simulink model "Control_Schematic_4"  (Simulink 8.3)
settings: Solver=FixedStepDiscrete  StartTime=0.0  StopTime=386.832  FixedStep=Ts  RelTol=1e-3
values from neighbouring files (symbols this model uses):
  B = [0 Kappa]'    [StartUp_5.m]    (also in StartUp_6.m)
  b = 156    [StartUp_10_Validation.m]    (also in StartUp_12.m; StartUp_12a.m; StartUp_2.m; StartUp_5.m)
  d = 13.52    [StartUp_10_Validation.m]    (also in StartUp_12.m; StartUp_12a.m; StartUp_2.m = 16.4; StartUp_5.m = 0.91)
  d0 = d*h    (= 0.328)    [StartUp_2.m]    (also in StartUp_5.m = 0.000455; StartUp_6.m = 0.000455)
  h = .02    (= 0.02)    [StartUp_2.m]    (also in StartUp_5.m = 0.0005; StartUp_6.m = 0.0005)
  K1 = .23    (= 0.23)    [StartUp_12.m]    (also in StartUp_12a.m; StartUp_2.m = PolyCon(1,2); StartUp_5.m = 16; StartUp_6.m = 16)
  K2 = .83    (= 0.83)    [StartUp_12.m]    (also in StartUp_12a.m; StartUp_2.m = 0.7; StartUp_5.m = 8; StartUp_6.m = 8)
  Kappa = (1E3/r)/((jw/r)+(m*r*.4))    (= 0.770469447034)    [StartUp_10_Validation.m]    (also in StartUp_12.m; StartUp_12a.m; StartUp_5.m = 0.000542967645047; StartUp_6.m = 0.000542967645047)
  Obz = c2d(Obs,Ts,'tustin')    [StartUp_2.m]    (also in StartUp_5.m; StartUp_6.m)
  P = [L(1,1) L(2,1);L(3,1) L(4,1)]    [StartUp_5.m]    (also in StartUp_6.m; charatioass.m = roots(K))
  r = 50    [StartUp_10_Validation.m]    (also in StartUp_12.m; StartUp_12a.m; StartUp_2.m = 820; StartUp_5.m = 0.01)
  R = 50    [StartUp_2.m]    (also in StartUp_5.m; StartUp_6.m)
  TD = ss(Atd,Btd,Ctd,Dtd,Ts)    [StartUp_12.m]    (also in StartUp_12a.m; StartUp_2.m; StartUp_5.m; StartUp_6.m)
  Ts = 1/100    (= 0.01)    [StartUp_10_Validation.m]    (also in StartUp_12.m; StartUp_12a.m; StartUp_2.m = 0.001; StartUp_5.m = 0.001)
undefined symbols (not defined in the file or in its folder): DiscIntNeverNeededParam, sigbuilder_block
undefined symbols (not defined in the file): ADAMS_cwd, ADAMS_exec, ADAMS_host, ADAMS_init, ADAMS_inputs, ADAMS_outputs, ADAMS_prefix, ADAMS_static, ADAMS_sysdir
libraries: simulink x1
settings Model: Creator=baqumau  LastModifiedBy=baqumau
settings DataIOCC: SignalLoggingSaveFormat=Dataset
settings DebuggingCC: UnderspecifiedInitializationDetection=Simplified  StateNameClashWarn=none
settings GRTTargetCC: CombineOutputUpdateFcns=on  GRTInterface=off

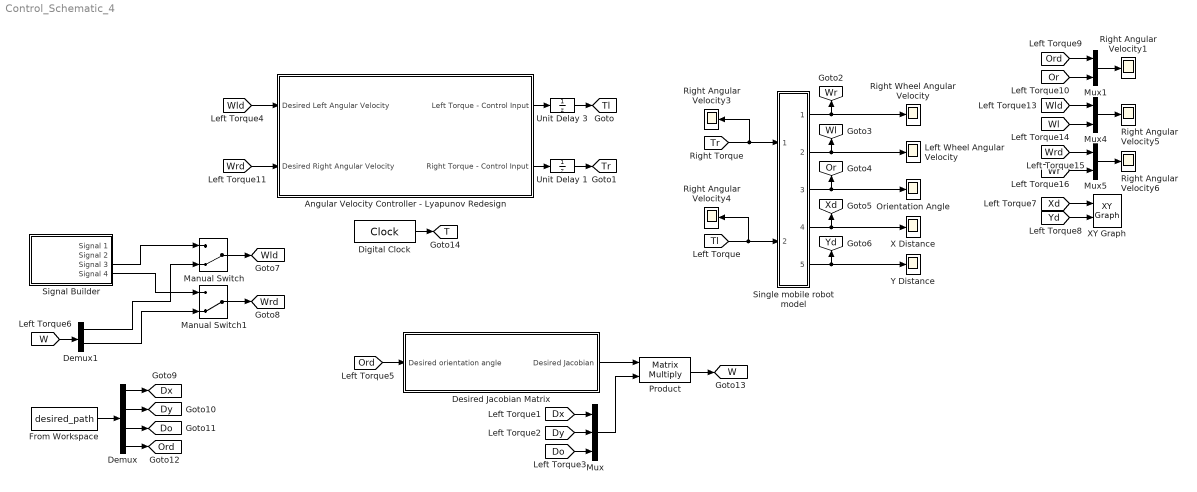
== system Control_Schematic_4 ==
  Angular Velocity Controller - Lyapunov Redesign : Subsystem
  Demux : Demux
  Demux1 : Demux  Outputs=2
  Desired Jacobian Matrix : Subsystem
  Digital Clock : DigitalClock  SampleTime=Ts
  From Workspace : FromWorkspace  VariableName=desired_path  SampleTime=Ts
  Left Wheel Angular Velocity : Scope
      settings: SaveName=ScopeData2
  Manual Switch : ManualSwitch  CurrentSetting=0
  Manual Switch1 : ManualSwitch  CurrentSetting=0
  Mux : Mux  Inputs=3
  Mux1 : Mux  Inputs=2
  Mux4 : Mux  Inputs=2
  Mux5 : Mux  Inputs=2
  Orientation Angle : Scope
      settings: YMin=-4  YMax=4
  Product : Product  Multiplication=Matrix(*)
  Right Angular Velocity{1,3..6} (5 alike) : Scope
      Right Angular Velocity1 settings: YMin=-3  YMax=3  SaveName=ScopeData27
      Right Angular Velocity3 settings: YMin=-25  YMax=25  SaveName=ScopeData7
      Right Angular Velocity4 settings: YMin=-25  YMax=25  SaveName=ScopeData8
      Right Angular Velocity5 settings: YMin=-1  YMax=1  SaveName=ScopeData9
      Right Angular Velocity6 settings: YMin=-1  YMax=3  SaveName=ScopeData10
  Right Wheel Angular Velocity : Scope
      settings: YMin=-1  YMax=1  SaveName=ScopeData3
  Signal Builder : Subsystem  Tag=STV Subsys  LoadFcn=sigbuilder_block('load');  StartFcn=sigbuilder_block('start');  StopFcn=sigbuilder_block('stop');  ClipboardFcn=sigbuilder_block('clipboard');  mask(Sigbuilder block){}
      mask help: Simulink:masks:SigbuilderBlock_MD
      mask init:
      | if ~strcmp(get_param(bdroot(gcbh),'SimulationStatus'),'stopped') tuvar = sigbuilder_block('maskInit'); end
      settings: CopyFcn=sigbuilder_block('copy');  DeleteFcn=sigbuilder_block('delete');  ModelCloseFcn=sigbuilder_block('modelClose');  PreSaveFcn=sigbuilder_block('preSave');  PauseFcn=sigbuilder_block('pause');  ContinueFcn=sigbuilder_block('continue');  NameChangeFcn=sigbuilder_block('namechange');  OpenFcn=sigbuilder_block('open',[437.25 118.5 550.5 394.5 ]);  CloseFcn=sigbuilder_block('close');
      mask Display: plot(0, 0, 100, 100,[2, 2, 32, 32, 2], [68, 8, 8, 68, 68],[32, 2], [38, 38], [32, 19, 2],[53, 60, 44], [32, 17, 17, 2],[16, 16, 31, 31]);txt = getActiveGroup(gcbh);text(2, 100, txt,'verticalAlignment', 'top');
  Single mobile robot model : Subsystem
  Unit Delay 1 : UnitDelay  SampleTime=-1
  Unit Delay 3 : UnitDelay  SampleTime=-1
  X Distance : Scope
      settings: YMin=0  YMax=2600  SaveName=ScopeData4
  XY Graph : simulink/Sinks/XY Graph  xmin=0  xmax=5000  ymin=0  ymax=5000  st=Ts
  Y Distance : Scope
      settings: YMin=0  YMax=1000
  tag scope: Do=global, Dx=global, Dy=global, Or=global, Ord=global, T=global, Tl=global, Tr=global, W=global, Wl=global, Wld=global, Wr=global, Wrd=global, Xd=global, Yd=global
  wires:
  Single mobile robot model/1(Wrw) -> Right Wheel Angular Velocity/1, [Wr]
  Single mobile robot model/2(Wlw) -> Left Wheel Angular Velocity/1, [Wl]
  Single mobile robot model/3(Alpha) -> Orientation Angle/1, [Or]
  Single mobile robot model/4(X_Dist) -> X Distance/1, [Xd]
  Single mobile robot model/5(Y_Dist) -> Y Distance/1, [Yd]
  [Tr] -> Single mobile robot model/1(Trw), Right Angular Velocity3/1
  [Tl] -> Single mobile robot model/2(Tlw), Right Angular Velocity4/1
  [Wld] -> Angular Velocity Controller - Lyapunov Redesign/1(Desired Left Angular Velocity)
  [Wrd] -> Angular Velocity Controller - Lyapunov Redesign/2(Desired Right Angular Velocity)
  [Wld] -> Mux4/1
  [Wl] -> Mux4/2
  Mux4/1 -> Right Angular Velocity5/1
  [Wrd] -> Mux5/1
  [Wr] -> Mux5/2
  Mux5/1 -> Right Angular Velocity6/1
  Manual Switch/1 -> [Wld]
  Manual Switch1/1 -> [Wrd]
  From Workspace/1 -> Demux/1
  Demux/1 -> [Dx]
  Demux/2 -> [Dy]
  Demux/3 -> [Do]
  Demux/4 -> [Ord]
  [Dy] -> Mux/2
  [Dx] -> Mux/1
  [Do] -> Mux/3
  [Ord] -> Desired Jacobian Matrix/1(Desired orientation angle)
  Desired Jacobian Matrix/1(Desired Jacobian) -> Product/1
  Mux/1 -> Product/2
  Product/1 -> [W]
  [W] -> Demux1/1
  Demux1/1 -> Manual Switch/2
  Demux1/2 -> Manual Switch1/2
  Signal Builder/3(Signal 3) -> Manual Switch/1
  Signal Builder/4(Signal 4) -> Manual Switch1/1
  [Xd] -> XY Graph/1
  [Yd] -> XY Graph/2
  Digital Clock/1 -> [T]
  [Ord] -> Mux1/1
  [Or] -> Mux1/2
  Mux1/1 -> Right Angular Velocity1/1
  Angular Velocity Controller - Lyapunov Redesign/1(Left Torque - Control Input) -> Unit Delay 3/1
  Angular Velocity Controller - Lyapunov Redesign/2(Right Torque - Control Input) -> Unit Delay 1/1
  Unit Delay 3/1 -> [Tl]
  Unit Delay 1/1 -> [Tr]

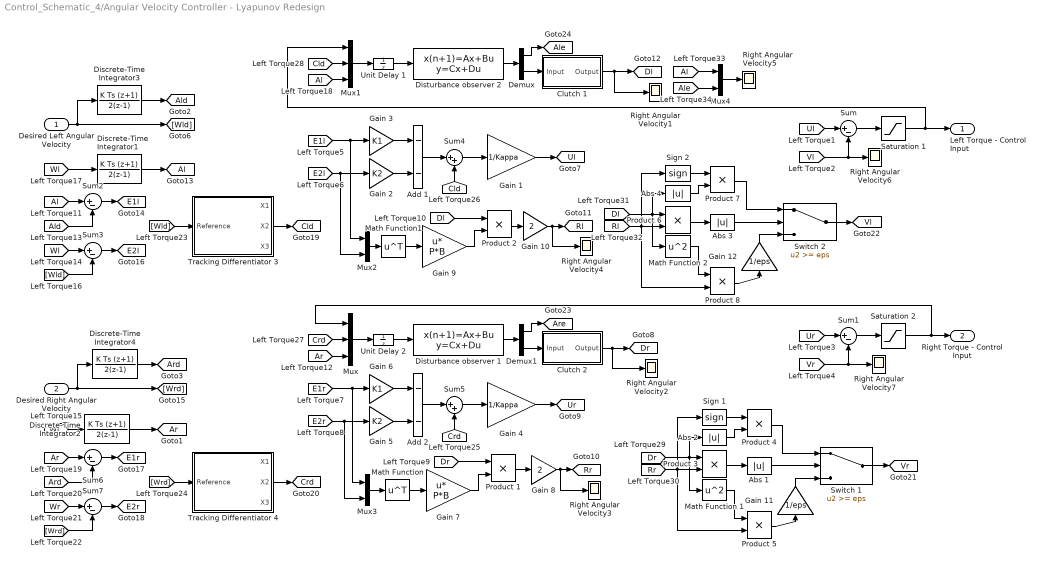
== system Control_Schematic_4/Angular Velocity Controller - Lyapunov Redesign ==
  Desired Left Angular Velocity : Inport
  Desired Right Angular Velocity : Inport  Port=2
  Abs {1..4} (4 alike) : Abs
  Add 1 : Sum  Inputs=--
  Add 2 : Sum  Inputs=--
  Clutch 1 : Subsystem
  Clutch 2 : Subsystem
  Demux : Demux  Outputs=2
  Demux1 : Demux  Outputs=2
  Discrete-Time Integrator{1..4} (4 alike) : DiscreteIntegrator  IntegratorMethod=Integration: Trapezoidal  gainval=1  SampleTime=Ts  ICPrevOutput=DiscIntNeverNeededParam  ICPrevScaledInput=DiscIntNeverNeededParam
  Disturbance observer 1 : DiscreteStateSpace  A=Obz.a  B=Obz.b  C=Obz.c  D=Obz.d  SampleTime=Ts
  Disturbance observer 2 : DiscreteStateSpace  A=Obz.a  B=Obz.b  C=Obz.c  D=Obz.d  SampleTime=Ts
  Gain 1 : Gain  Gain=1/Kappa
  Gain 10 : Gain  Gain=2
  Gain 11 : Gain  Gain=1/eps
  Gain 12 : Gain  Gain=1/eps
  Gain 2 : Gain  Gain=K2
  Gain 3 : Gain  Gain=K1
  Gain 4 : Gain  Gain=1/Kappa
  Gain 5 : Gain  Gain=K2
  Gain 6 : Gain  Gain=K1
  Gain 7 : Gain  Gain=P*B  Multiplication=Matrix(u*K)
  Gain 8 : Gain  Gain=2
  Gain 9 : Gain  Gain=P*B  Multiplication=Matrix(u*K)
  Math Function : Math  Operator=transpose  SaturateOnIntegerOverflow=on
  Math Function 1 : Math  Operator=square  SaturateOnIntegerOverflow=on
  Math Function 2 : Math  Operator=square  SaturateOnIntegerOverflow=on
  Math Function1 : Math  Operator=transpose  SaturateOnIntegerOverflow=on
  Mux : Mux  Inputs=3
  Mux1 : Mux  Inputs=3
  Mux2 : Mux  Inputs=2
  Mux3 : Mux  Inputs=2
  Mux4 : Mux  Inputs=2
  Product {1..8} (8 alike) : Product
  Right Angular Velocity{1..7} (7 alike) : Scope
      Right Angular Velocity1 settings: YMin=-3  YMax=3  SaveName=ScopeData5
      Right Angular Velocity2 settings: YMin=-3  YMax=3  SaveName=ScopeData6
      Right Angular Velocity3 settings: YMin=-3  YMax=3  SaveName=ScopeData11
      Right Angular Velocity4 settings: YMin=-3  YMax=3  SaveName=ScopeData12
      Right Angular Velocity5 settings: YMin=-1  YMax=1  SaveName=ScopeData13
      Right Angular Velocity6 settings: YMin=-3  YMax=3  SaveName=ScopeData14
      Right Angular Velocity7 settings: YMin=-3  YMax=3  SaveName=ScopeData15
  Saturation 1 : Saturate  UpperLimit=20  LowerLimit=-20
  Saturation 2 : Saturate  UpperLimit=20  LowerLimit=-20
  Sign 1 : Signum
  Sign 2 : Signum
  Sum{,1..3,6..7} (6 alike) : Sum  Inputs=|+-
  Sum4 : Sum  Inputs=|++
  Sum5 : Sum  Inputs=|++
  Switch 1 : Switch  Threshold=eps
  Switch 2 : Switch  Threshold=eps
  Tracking Differentiator 3 : Subsystem
  Tracking Differentiator 4 : Subsystem
  Unit Delay 1 : UnitDelay  SampleTime=-1
  Unit Delay 2 : UnitDelay  SampleTime=-1
  Left Torque - Control Input : Outport
  Right Torque - Control Input : Outport  Port=2
  tag scope: Al=global, Ald=global, Ale=global, Ar=global, Ard=global, Are=global, Cld=global, Crd=global, Dl=global, Dr=global, E1l=global, E1r=global, E2l=global, E2r=global, Rl=global, Rr=global, Ul=global, Ur=global, Vl=global, Vr=global
  wires:
  Discrete-Time Integrator1/1 -> [Al]
  Discrete-Time Integrator2/1 -> [Ar]
  Saturation 1/1 -> Mux1/1, Left Torque - Control Input/1
  Saturation 2/1 -> Mux/1, Right Torque - Control Input/1
  Discrete-Time Integrator4/1 -> [Ard]
  Discrete-Time Integrator3/1 -> [Ald]
  [Wl] -> Discrete-Time Integrator1/1
  [Wr] -> Discrete-Time Integrator2/1
  Mux/1 -> Unit Delay 2/1
  Mux1/1 -> Unit Delay 1/1
  Sum/1 -> Saturation 1/1
  Sum1/1 -> Saturation 2/1
  [Ul] -> Sum/1
  [Ur] -> Sum1/1
  Gain 3/1 -> Add 1/1
  Gain 2/1 -> Add 1/2
  Gain 1/1 -> [Ul]
  Gain 6/1 -> Add 2/1
  Gain 5/1 -> Add 2/2
  [E1r] -> Mux3/1, Gain 6/1
  [E2r] -> Mux3/2, Gain 5/1
  Gain 4/1 -> [Ur]
  [Dr] -> Product 1/1
  Mux3/1 -> Math Function/1
  [E1l] -> Mux2/1, Gain 3/1
  [E2l] -> Mux2/2, Gain 2/1
  [Al] -> Sum2/1
  [Ald] -> Sum2/2
  Sum2/1 -> [E1l]
  [Wl] -> Sum3/1
  [Wld] -> Sum3/2
  Sum3/1 -> [E2l]
  Sum4/1 -> Gain 1/1
  Sum5/1 -> Gain 4/1
  [Ar] -> Sum6/1
  [Ard] -> Sum6/2
  Sum6/1 -> [E1r]
  [Wr] -> Sum7/1
  [Wrd] -> Sum7/2
  Sum7/1 -> [E2r]
  Add 2/1 -> Sum5/1
  Add 1/1 -> Sum4/1
  [Wld] -> Tracking Differentiator 3/1(Reference)
  Tracking Differentiator 3/2(X2) -> [Cld]
  [Wrd] -> Tracking Differentiator 4/1(Reference)
  Tracking Differentiator 4/2(X2) -> [Crd]
  [Ar] -> Mux/3
  [Crd] -> Mux/2
  [Al] -> Mux1/3
  [Cld] -> Mux1/2
  [Dr] -> Math Function 1/1, Abs 2/1, Product 3/1
  [Rr] -> Product 5/2, Sign 1/1, Product 3/2
  Product 3/1 -> Abs 1/1
  Abs 1/1 -> Switch 1/2
  Switch 1/1 -> [Vr]
  Sign 1/1 -> Product 4/1
  Abs 2/1 -> Product 4/2
  Product 4/1 -> Switch 1/1
  Math Function 1/1 -> Product 5/1
  Product 5/1 -> Gain 11/1
  Gain 11/1 -> Switch 1/3
  [Dl] -> Product 6/1, Abs 4/1, Math Function 2/1
  [Rl] -> Product 6/2, Sign 2/1, Product 8/2
  Product 6/1 -> Abs 3/1
  Abs 3/1 -> Switch 2/2
  Switch 2/1 -> [Vl]
  Sign 2/1 -> Product 7/1
  Abs 4/1 -> Product 7/2
  Product 7/1 -> Switch 2/1
  Math Function 2/1 -> Product 8/1
  Product 8/1 -> Gain 12/1
  Gain 12/1 -> Switch 2/3
  Math Function/1 -> Gain 7/1
  Gain 7/1 -> Product 1/2
  Product 1/1 -> Gain 8/1
  Gain 8/1 -> Right Angular Velocity3/1, [Rr]
  [Dl] -> Product 2/1
  Math Function1/1 -> Gain 9/1
  Gain 9/1 -> Product 2/2
  Product 2/1 -> Gain 10/1
  Mux2/1 -> Math Function1/1
  Unit Delay 1/1 -> Disturbance observer 2/1
  Unit Delay 2/1 -> Disturbance observer 1/1
  Gain 10/1 -> Right Angular Velocity4/1, [Rl]
  Clutch 1/1(Output) -> Right Angular Velocity1/1, [Dl]
  Clutch 2/1(Output) -> Right Angular Velocity2/1, [Dr]
  Disturbance observer 2/1 -> Demux/1
  Demux/2 -> Clutch 1/1(Input)
  Disturbance observer 1/1 -> Demux1/1
  Demux1/2 -> Clutch 2/1(Input)
  Demux1/1 -> [Are]
  Demux/1 -> [Ale]
  [Ale] -> Mux4/2
  Mux4/1 -> Right Angular Velocity5/1
  [Al] -> Mux4/1
  [Vr] -> Right Angular Velocity7/1, Sum1/2
  [Vl] -> Right Angular Velocity6/1, Sum/2
  [Cld] -> Sum4/2
  [Crd] -> Sum5/2
  Desired Left Angular Velocity/1 -> [Wld], Discrete-Time Integrator3/1
  Desired Right Angular Velocity/1 -> [Wrd], Discrete-Time Integrator4/1

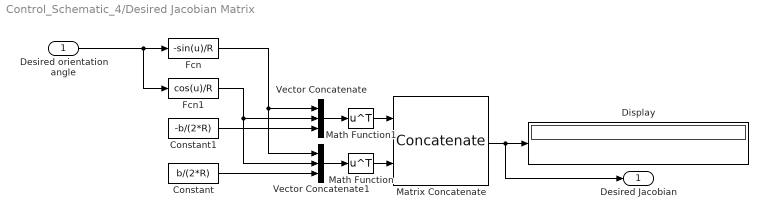
== system Control_Schematic_4/Desired Jacobian Matrix ==
  Desired orientation angle : Inport
  Constant : Constant  Value=b/(2*R)
  Constant1 : Constant  Value=-b/(2*R)
  Display : Display
  Fcn : Fcn  Expr=-sin(u)/R
  Fcn1 : Fcn  Expr=cos(u)/R
  Math Function : Math  Operator=transpose  SaturateOnIntegerOverflow=on
  Math Function1 : Math  Operator=transpose  SaturateOnIntegerOverflow=on
  Matrix Concatenate : Concatenate  Mode=Multidimensional array
  Vector Concatenate : Concatenate  NumInputs=3
  Vector Concatenate1 : Concatenate  NumInputs=3
  Desired Jacobian : Outport
  wires:
  Math Function/1 -> Matrix Concatenate/2
  Math Function1/1 -> Matrix Concatenate/1
  Desired orientation angle/1 -> Fcn1/1, Fcn/1
  Constant1/1 -> Vector Concatenate/3
  Matrix Concatenate/1 -> Desired Jacobian/1, Display/1
  Fcn/1 -> Vector Concatenate1/1, Vector Concatenate/1
  Vector Concatenate/1 -> Math Function1/1
  Fcn1/1 -> Vector Concatenate1/2, Vector Concatenate/2
  Constant/1 -> Vector Concatenate1/3
  Vector Concatenate1/1 -> Math Function/1

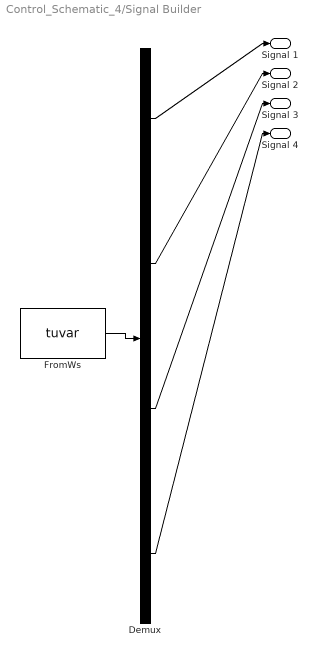
== system Control_Schematic_4/Signal Builder ==
  Demux : Demux  Tag=STV Demux
  FromWs : FromWorkspace  Tag=STV FromWs  VariableName=tuvar  SampleTime=0  SigBuilderData=DataTag0  VnvData=DataTag1
      SigBuilderData=|
      | common.afterFinalStr = 'Extrapolate'
      | common.sampleTime = 0
      | dataSet.timeRange = [0 10]
      | dataSet.name = 'Group 1'
      | sbobj.Groups.Name = 'Group 1'
      | sbobj.Groups.Signals(1).Name = 'Signal 1'
      | sbobj.Groups.Signals(1).XData = [0 1 2 3 4 5 6 7 8 8 9 10]
      | sbobj.Groups.Signals(1).YData = [0 1.5 2.05 1.54 0.9 0 -1.58 -2.05 -1.65 -1.66 0 0.85]
      | sbobj.Groups.Signals(2).Name = 'Signal 2'
      | sbobj.Groups.Signals(2).XData = [0 1 2 2 3 4 4 5 6 7 8 9 10]
      | sbobj.Groups.Signals(2).YData = [0 -1 -1.35 -1.3 -2 -2 -2.05 -0.6 2 2 1.5 -1.15 -2.85]
      | sbobj.Groups.Signals(3).Name = 'Signal 3'
      | sbobj.Groups.Signals(3).XData = [0 10]
      | sbobj.Groups.Signals(3).YData = [1.28205128205 1.28205128205]
      | sbobj.Groups.Signals(4).Name = 'Signal 4'
      | sbobj.Groups.Signals(4).XData = [0 10]
      | sbobj.Groups.Signals(4).YData = [0 0]
  Signal 1 : Outport  Tag=STV Outport
  Signal 2 : Outport  Tag=STV Outport  Port=2
  Signal 3 : Outport  Tag=STV Outport  Port=3
  Signal 4 : Outport  Tag=STV Outport  Port=4
  wires:
  FromWs/1 -> Demux/1
  Demux/1 -> Signal 1/1
  Demux/2 -> Signal 2/1
  Demux/3 -> Signal 3/1
  Demux/4 -> Signal 4/1

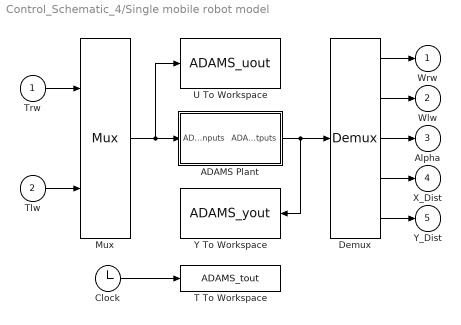
== system Control_Schematic_4/Single mobile robot model ==
  Trw : Inport
  Tlw : Inport  Port=2
  ADAMS Plant : Subsystem  LoadFcn=|  InitFcn=clear mex  mask(Adams Plant){exevie=ADAMS_sysdir, nam_in=ADAMS_inputs, namout=ADAMS_outputs, nampre=ADAMS_prefix, outfil=ADAMS_prefix, exesol=ADAMS_exec, stat=ADAMS_static, inicmd=[ADAMS_init], exetyp=C++, comtyp=PIPE(DDE), workdir=ADAMS_cwd, ada_host=ADAMS_host, modani=batch, modsim=discrete, dft=no, simulink_lead_cosim=yes, pin_interp_order=0, pout_extrap_order=0, pin_extrap_order=0, pout_interp_order=0, dt_out=Ts, o_rate=1, more=off}
      | %check based on dialog box setting for when setting by popup menu                                             
      | if exist('ADAMS_solver_type')                                                                                 
      |   if strcmp(ADAMS_solver_type,'C++')                                                                          
      |     set_param(gcb,'exetyp','C++');                                                                            
      |   else                                                                                                        
      |     set_param(gcb,'exetyp','Fortran');                                                                        
      |   end                                                                                                         
      | else                                                                                                          
      |   set_param(gcb,'exetyp','C++');                                                                              
      | end                                                                                                           
      | %set the mode if using acar_solver                                                                            
      | %REQUIRED HERE BECAUSE BELOW CAUSES MDLTERMINATE TO BE CALLED 2 TIMES IN MIDDLE OF SIMULATION WHEN SET IN MASK
      |                                                                                                               
      | %enable the direct feedthrough, sim mode, anim mode parameters by default                                     
      |                                                                                                               
      | if exist('set_some_params_states')                                                                            
      |                                                                                                               
      |   set_some_params_states({'dft','modsim','modani'},{'on','on','on'},'MaskEnables',gcb)                        
      |   %turn on direct feedthrough option                                                                          
      |   set_some_params_states({'dft'},{'on'},'MaskVisibilities',gcb)                                               
      |                                                                                                               
      |  end                                                                                                          
      |                                                                                                               
      |                                                                                                               
      | if exist('ADAMS_exec')                                                                                        
      |   if and(strcmp(get_param(gcb,'exesol'),'ADAMS_exec'),strcmp(ADAMS_exec,'acar_solver'))                       
      |     %set the sim mode to discrete -- only supported mode                                                      
      |     set_param(gcb,'modsim','discrete')                                                                        
      |      %turn off direct feedthrough option                                                                      
      |      set_some_params_states({'dft'},{'off'},'MaskVisibilities',gcb)                                           
      |     %set the animation mode to batch -- only supported mode                                                   
      |     set_param(gcb,'modani','batch')                                                                           
      |     %disable the direct feedthrough, sim mode, anim mode parameters                                           
      |     set_some_params_states({'modsim','modani'},{'off','off'},'MaskEnables',gcb)                               
      |   end                                                                                                         
      | end
      mask prompts: exevie "Adams install directory"; nam_in "Adams/View input names"; namout "Adams/View output names"; nampre "Adams model file prefix"; outfil "Output files prefix (opt.: if blank - no output)"; exesol "User executable (opt.: if blank - use standard)"; stat "Initial static simulation flag"; inicmd "Initialization commands"; exetyp "Adams/Solver type"; comtyp "Interprocess option"; workdir "Adams working directory"; ada_host "Adams host"; modani "Animation mode"; modsim "Simulation mode"; dft "Direct feedthrough"; simulink_lead_cosim "Discrete Computational Order - Simulink Leads Adams"; pin_interp_order "Plant input interpolation order"; pout_extrap_order "Plant output extrapolation order"; pin_extrap_order "Plant input extrapolation order"; pout_interp_order "Plant output interpolation order"; dt_out "Communication interval"; o_rate "Number of communications per output step"; more "More parameters"
      mask help: Simulate any Adams plant model either in Adams/Solver form (.adm file) or in Adams/View form (.cmd file)
      settings: OpenFcn=|
      | open_system(gcb,'mask')
      | if not(exist('set_some_params_states'))
      | 
      | warning('The script "set_some_params_states.m" cannot be found in the MATLAB PATH.  Cannot update the ADAMS Plant S-Function parameters.')
      | 
      | warning('Recommended action(optional):  run the Adams/Controls .m file first to help choose the correct settings in the Adams S-Function block.')
      | 
      | end
      mask Help:
      | <html>
      | This S-Function represents the non-linear Adams Plant with the inputs sent to the Adams model <br>
      |  and the outputs generated by the Adams model.  See the Adams/Controls documentation for more <br>
      | information.  This plant uses the following variables:<br>
      | <br>
      | <b>ADAMS_sysdir  :</b> Adams installation directory<br>
      | <b>ADAMS_inputs  :</b> Input variables View names vector<br>
      | <b>ADAMS_outputs :</b> Outputs variables View names vector<br>
      | <b>ADAMS_prefix  : </b>ADAMS model files prefix (.adm, .cmd); also doubles as output files prefix<br>
      | <b>ADAMS_exec :</b> Adams/Solver user library or keyword (e.g., acar_solver)<br>
      | <b>ADAMS_static :</b> yes|no - initial static before Co-simulation(discrete)/Function Evaluation(continuous)<br>
      | <b>ADAMS_init :</b>Initialization commands (i.e., Adams/View or Solver commands, depending on setting for Animation mode)<br>
      | <b>ADAMS_cwd : </b> Current working directory (for TCP/IP)<br>
      | <b>ADAMS_host : </b>Name of Adams server host (for TCP/IP)<br>
      | <b>ADAMS_mode :</b> Linear or non-linear (i.e., co-sim, function eval)<br>
      | <b>ADAMS_solver_type :</b>Fortran or C++ (used to set popup menu when first loaded) <br>
      | 
      | 
      | <br>
      | The following settings can be chosen:<br>
      | <br>
      | <b>Adams/Solver type:</b>  Fortran or C++ (will also set ADAMS_solver_type)<br>
      | <b>Interprocess option:</b> Pipe(DDE) or TCP/IP; TCP/IP can allow different machines run Adams and MATLAB<br>
      | <b>Animation mode:</b> batch (Solver, uses .adm) or interactive (View, uses .cmd)<br>
      | <b>Simulation mode:</b> discrete (Co-simulation) or continuous (Function Evaluation)<br>
      | <b>Discrete Computational Order - Simulink Lead Adams:</b> for discrete mode, chooses if Simulink leads the integration (yes) or lags (no);<br> if set to "no", can remove algebraic loop<br>
      | <b>Plant input interpolation order:</b> 0 = zero-order hold; 1 = linear (discrete mode only, where Simulink leads)<br>
      | <b>Plant output extrapolation order:</b> 0 = zero-order hold;1 = linear(discrete mode only, where Simulink leads)<br>
      | <b>Plant input extrapolation order:</b> 0 = zero-order hold; 1 = linear (discrete mode only, where Adams leads)<br>
      | <b>Plant output interpolation order:</b> 0 = zero-order hold;1 = linear(discrete mode only, where Adams leads)<br>
      | <b>Direct feedthrough:</b> yes|no - yes = Input directly effect output(continuous mode-only)<br>
      | <b>Communication interval:</b> Time step at which Co-simulation exchange information (e.g.,0.005); also controls <br>output for continuous mode (Function Evaluation)<br>
      | <b>Number of communications per output step: </b>Sets Adams output rate (.res, .req, .gra) integer value (default: 1)<br>
      | </html>
      mask Callback exesol:
      | if exist('set_some_params_states')
      | %enable the direct feedthrough, sim mode, anim mode parameters
      | set_some_params_states({'dft','modsim','modani'},{'on','on','on'},'MaskEnables',gcb)
      | %turn on direct feedthrough option
      | set_some_params_states({'dft'},{'on'},'MaskVisibilities',gcb)
      | end
      | 
      | if exist('ADAMS_exec')
      |   if and(strcmp(get_param(gcb,'exesol'),'ADAMS_exec'),strcmp(ADAMS_exec,'acar_solver'))
      |     %set the sim mode to discrete -- only supported mode
      |     %REMOVED:  BELOW CAUSES MDLTERMINATE TO BE CALLED 2 TIMES IN MIDDLE OF SIMULATION
      |     %Now in LoadFcn callback
      |     %set_param(gcb,'modsim','discrete')
      |      %turn off direct feedthrough option
      |     set_some_params_states({'dft'},{'off'},'MaskVisibilities',gcb)
      |     %set the animation mode to batch -- only supported mode
      |     %REMOVED:  BELOW CAUSES MDLTERMINATE TO BE CALLED 2 TIMES IN MIDDLE OF SIMULATION
      |     %Now in LoadFcn callback
      |     %set_param(gcb,'modani','batch')
      |     %disable the direct feedthrough, sim mode, anim mode parameters
      |     set_some_params_states({'modsim','modani'},{'off','off'},'MaskEnables',gcb)
      |   end
      | end
      mask TypeOptions exetyp: Fortran | C++
      mask Callback exetyp:
      | if strcmp(get_param(gcb,'exetyp'),'C++')
      |     ADAMS_solver_type='C++';
      | else
      |     ADAMS_solver_type='Fortran';
      | end
      mask TypeOptions comtyp: PIPE(DDE) | TCP/IP
      mask Callback comtyp:
      | if exist('set_some_params_states')
      | if strcmp(get_param(gcb,'comtyp'),'PIPE(DDE)')
      |     %turn off cwd, host options
      |     set_some_params_states({'ada_host','workdir'},{'off','off'},'MaskVisibilities',gcb)
      | else%if strcmp(get_param(gcb,'modsim'),'TCP/IP')
      |     %turn on cwd, host options
      |     set_some_params_states({'ada_host','workdir'},{'on','on'},'MaskVisibilities',gcb)
      | end
      | end
      mask TypeOptions modani: batch | interactive
      mask TypeOptions modsim: discrete | continuous
      mask Callback modsim:
      | if exist('set_some_params_states')
      | if strcmp(get_param(gcb,'modsim'),'discrete')
      |      %turn off direct feedthrough option
      |     set_some_params_states({'dft'},{'off'},'MaskVisibilities',gcb)
      |     %turn on discrete co-sim type if want to see more
      |     if strcmp(get_param(gcb,'more'),'on')
      |         set_some_params_states({'simulink_lead_cosim'},{'on'},'MaskVisibilities',gcb)
      |     end
      |     if strcmp(get_param(gcb,'simulink_lead_cosim'),'yes')
      |         %turn on interpolation/extrapolation options
      |         set_some_params_states({'pin_interp_order','pout_extrap_order',},{'on','on'},'MaskVisibilities',gcb)
      |     else
      |         set_some_params_states({'pin_extrap_order','pout_interp_order'},{'on','on'},'MaskVisibilities',gcb)
      |     end
      | else%if strcmp(get_param(gcb,'modsim'),'continuous')
      |      %turn off direct feedthrough option
      |     set_some_params_states({'dft'},{'on'},'MaskVisibilities',gcb)
      |     %turn off interpolation/extrapolation options
      |     set_some_params_states({'pin_interp_order','pout_extrap_order','pin_extrap_order','pout_interp_order','simulink_lead_cosim'},{'off','off','off','off','off'},'MaskVisibilities',gcb)
      | end
      | end
      mask TypeOptions dft: no | yes
      mask TypeOptions simulink_lead_cosim: yes | no
      mask Callback simulink_lead_cosim:
      | if exist('set_some_params_states')
      | if (strcmp(get_param(gcb,'simulink_lead_cosim'),'yes') && strcmp(get_param(gcb,'modsim'),'discrete'))
      |      %turn off unused interpolate/extrapolate options
      |     set_some_params_states({'pin_extrap_order','pout_interp_order'},{'off','off'},'MaskVisibilities',gcb)
      |     %turn on used interpolate/extrapolate options
      |     set_some_params_states({'pin_interp_order','pout_extrap_order'},{'on','on'},'MaskVisibilities',gcb)
      | elseif (strcmp(get_param(gcb,'simulink_lead_cosim'),'no') && strcmp(get_param(gcb,'modsim'),'discrete'))
      |     %turn on used interpolate/extrapolate options
      |     set_some_params_states({'pin_extrap_order','pout_interp_order'},{'on','on'},'MaskVisibilities',gcb)
      |      %turn off unused interpolate/extrapolate options
      |     set_some_params_states({'pin_interp_order','pout_extrap_order'},{'off','off'},'MaskVisibilities',gcb)
      | end
      | end
      mask TypeOptions pin_interp_order: 0 | 1
      mask TypeOptions pout_extrap_order: 0 | 1
      mask TypeOptions pin_extrap_order: 0 | 1
      mask TypeOptions pout_interp_order: 0 | 1
      mask Callback more:
      | if exist('set_some_params_states')
      | if (strcmp(get_param(gcb,'more'),'on'))
      |      %turn on infrequently used options
      |     set_some_params_states({'exevie','nam_in','namout','exesol','stat','inicmd'},{'on','on','on','on','on','on'},'MaskVisibilities',gcb)
      |     if strcmp(get_param(gcb,'modsim'),'discrete')
      |         set_some_params_states({'simulink_lead_cosim'},{'on'},'MaskVisibilities',gcb)
      |     end
      | elseif (strcmp(get_param(gcb,'more'),'off'))
      |     %turn off infrequently used options
      |     set_some_params_states({'exevie','nam_in','namout','exesol','stat','inicmd'},{'off','off','off','off','off','off'},'MaskVisibilities',gcb)
      |     if strcmp(get_param(gcb,'modsim'),'discrete')
      |         set_some_params_states({'simulink_lead_cosim'},{'off'},'MaskVisibilities',gcb)
      |     end
      | end
      | end
      mask Display: disp( 'MSC Software' )
  Clock : Clock
  Demux : Demux  Outputs=5
  Mux : Mux  Inputs=2
  T To Workspace : ToWorkspace  VariableName=ADAMS_tout
      settings: MaxDataPoints=100000
  U To Workspace : ToWorkspace  VariableName=ADAMS_uout
      settings: MaxDataPoints=100000
  Y To Workspace : ToWorkspace  VariableName=ADAMS_yout
      settings: MaxDataPoints=100000
  Wrw : Outport
  Wlw : Outport  Port=2
  Alpha : Outport  Port=3
  X_Dist : Outport  Port=4
  Y_Dist : Outport  Port=5
  wires:
  Tlw/1 -> Mux/2
  Trw/1 -> Mux/1
  Demux/5 -> Y_Dist/1
  Demux/4 -> X_Dist/1
  Demux/3 -> Alpha/1
  Demux/2 -> Wlw/1
  Demux/1 -> Wrw/1
  ADAMS Plant/1(ADAMS outputs) -> Y To Workspace/1, Demux/1
  Mux/1 -> U To Workspace/1, ADAMS Plant/1(ADAMS inputs)
  Clock/1 -> T To Workspace/1

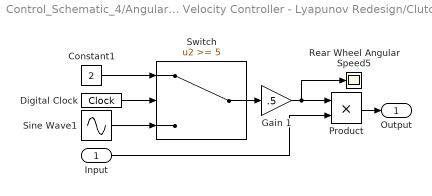
== system Control_Schematic_4/Angular Velocity Controller - Lyapunov Redesign/Clutch 1 ==
  Input : Inport
  Constant1 : Constant  Value=2
  Digital Clock : DigitalClock  SampleTime=Ts
  Gain 1 : Gain  Gain=.5
  Product : Product
  Rear Wheel Angular Speed5 : Scope
      settings: YMin=0  YMax=2  SaveName=ScopeData5
  Sine Wave1 : Sin  Bias=1  Frequency=(pi/5)  Phase=-pi/2  SampleTime=Ts
  Switch : Switch  Threshold=5
  Output : Outport
  wires:
  Constant1/1 -> Switch/1
  Digital Clock/1 -> Switch/2
  Switch/1 -> Gain 1/1
  Input/1 -> Product/2
  Product/1 -> Output/1
  Sine Wave1/1 -> Switch/3
  Gain 1/1 -> Rear Wheel Angular Speed5/1, Product/1

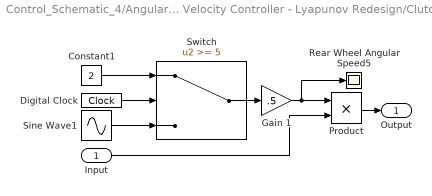
== system Control_Schematic_4/Angular Velocity Controller - Lyapunov Redesign/Clutch 2 ==
  Input : Inport
  Constant1 : Constant  Value=2
  Digital Clock : DigitalClock  SampleTime=Ts
  Gain 1 : Gain  Gain=.5
  Product : Product
  Rear Wheel Angular Speed5 : Scope
      settings: YMin=0  YMax=2  SaveName=ScopeData5
  Sine Wave1 : Sin  Bias=1  Frequency=(pi/5)  Phase=-pi/2  SampleTime=Ts
  Switch : Switch  Threshold=5
  Output : Outport
  wires:
  Gain 1/1 -> Product/1, Rear Wheel Angular Speed5/1
  Sine Wave1/1 -> Switch/3
  Product/1 -> Output/1
  Input/1 -> Product/2
  Switch/1 -> Gain 1/1
  Digital Clock/1 -> Switch/2
  Constant1/1 -> Switch/1

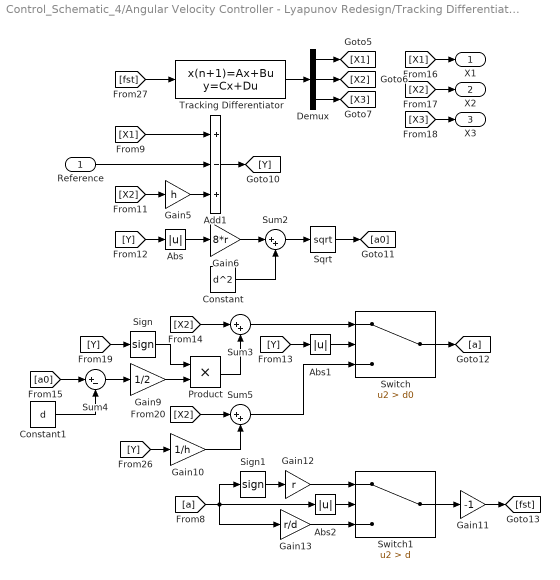
== system Control_Schematic_4/Angular Velocity Controller - Lyapunov Redesign/Tracking Differentiator 3 ==
  Reference : Inport
  Abs : Abs
  Abs1 : Abs
  Abs2 : Abs
  Add1 : Sum  Inputs=+-+
  Constant : Constant  Value=d^2
  Constant1 : Constant  Value=d
  Demux : Demux  Outputs=3
  Gain10 : Gain  Gain=1/h
  Gain11 : Gain  Gain=-1
  Gain12 : Gain  Gain=r
  Gain13 : Gain  Gain=r/d
  Gain5 : Gain  Gain=h
  Gain6 : Gain  Gain=8*r
  Gain9 : Gain  Gain=1/2
  Product : Product
  Sign : Signum
  Sign1 : Signum
  Sqrt : Sqrt  SaturateOnIntegerOverflow=on
  Sum2 : Sum  Inputs=|++
  Sum3 : Sum  Inputs=|++
  Sum4 : Sum  Inputs=|+-
  Sum5 : Sum  Inputs=|++
  Switch : Switch  Criteria=u2 > Threshold  Threshold=d0
  Switch1 : Switch  Criteria=u2 > Threshold  Threshold=d
  Tracking Differentiator : DiscreteStateSpace  A=TD.a  B=TD.b  C=TD.c  D=TD.d  SampleTime=Ts
  X1 : Outport
  X2 : Outport  Port=2
  X3 : Outport  Port=3
  wires:
  [X3] -> X3/1
  Gain5/1 -> Add1/3
  [X1] -> Add1/1
  Gain12/1 -> Switch1/1
  [X2] -> X2/1
  [X2] -> Gain5/1
  Reference/1 -> Add1/2
  [X1] -> X1/1
  Add1/1 -> [Y]
  Demux/1 -> [X1]
  Demux/3 -> [X3]
  Tracking Differentiator/1 -> Demux/1
  Demux/2 -> [X2]
  [Y] -> Abs/1
  Gain6/1 -> Sum2/1
  Abs/1 -> Gain6/1
  Constant/1 -> Sum2/2
  Sqrt/1 -> [a0]
  Sum2/1 -> Sqrt/1
  Abs1/1 -> Switch/2
  Sign1/1 -> Gain12/1
  Gain9/1 -> Product/2
  [Y] -> Abs1/1
  Sum3/1 -> Switch/1
  [X2] -> Sum3/1
  Sum4/1 -> Gain9/1
  Gain13/1 -> Switch1/3
  [a0] -> Sum4/1
  Product/1 -> Sum3/2
  Sign/1 -> Product/1
  Constant1/1 -> Sum4/2
  [X2] -> Sum5/1
  [fst] -> Tracking Differentiator/1
  Gain10/1 -> Sum5/2
  [a] -> Gain13/1, Sign1/1, Abs2/1
  Switch1/1 -> Gain11/1
  [Y] -> Sign/1
  Switch/1 -> [a]
  Sum5/1 -> Switch/3
  [Y] -> Gain10/1
  Abs2/1 -> Switch1/2
  Gain11/1 -> [fst]

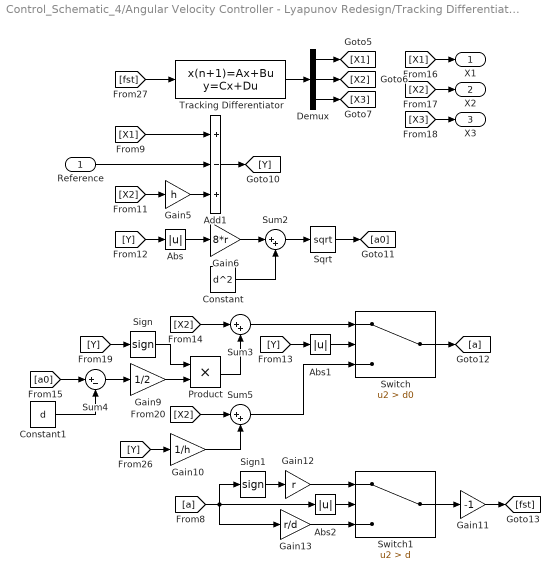
== system Control_Schematic_4/Angular Velocity Controller - Lyapunov Redesign/Tracking Differentiator 4 ==
  Reference : Inport
  Abs : Abs
  Abs1 : Abs
  Abs2 : Abs
  Add1 : Sum  Inputs=+-+
  Constant : Constant  Value=d^2
  Constant1 : Constant  Value=d
  Demux : Demux  Outputs=3
  Gain10 : Gain  Gain=1/h
  Gain11 : Gain  Gain=-1
  Gain12 : Gain  Gain=r
  Gain13 : Gain  Gain=r/d
  Gain5 : Gain  Gain=h
  Gain6 : Gain  Gain=8*r
  Gain9 : Gain  Gain=1/2
  Product : Product
  Sign : Signum
  Sign1 : Signum
  Sqrt : Sqrt  SaturateOnIntegerOverflow=on
  Sum2 : Sum  Inputs=|++
  Sum3 : Sum  Inputs=|++
  Sum4 : Sum  Inputs=|+-
  Sum5 : Sum  Inputs=|++
  Switch : Switch  Criteria=u2 > Threshold  Threshold=d0
  Switch1 : Switch  Criteria=u2 > Threshold  Threshold=d
  Tracking Differentiator : DiscreteStateSpace  A=TD.a  B=TD.b  C=TD.c  D=TD.d  SampleTime=Ts
  X1 : Outport
  X2 : Outport  Port=2
  X3 : Outport  Port=3
  wires:
  Gain11/1 -> [fst]
  Abs2/1 -> Switch1/2
  [Y] -> Gain10/1
  Sum5/1 -> Switch/3
  Switch/1 -> [a]
  [Y] -> Sign/1
  Switch1/1 -> Gain11/1
  [a] -> Abs2/1, Sign1/1, Gain13/1
  Gain10/1 -> Sum5/2
  [fst] -> Tracking Differentiator/1
  [X2] -> Sum5/1
  Constant1/1 -> Sum4/2
  Sign/1 -> Product/1
  Product/1 -> Sum3/2
  [a0] -> Sum4/1
  Gain13/1 -> Switch1/3
  Sum4/1 -> Gain9/1
  [X2] -> Sum3/1
  Sum3/1 -> Switch/1
  [Y] -> Abs1/1
  Gain9/1 -> Product/2
  Sign1/1 -> Gain12/1
  Abs1/1 -> Switch/2
  Sum2/1 -> Sqrt/1
  Sqrt/1 -> [a0]
  Constant/1 -> Sum2/2
  Abs/1 -> Gain6/1
  Gain6/1 -> Sum2/1
  [Y] -> Abs/1
  Demux/2 -> [X2]
  Tracking Differentiator/1 -> Demux/1
  Demux/3 -> [X3]
  Demux/1 -> [X1]
  Add1/1 -> [Y]
  [X1] -> X1/1
  Reference/1 -> Add1/2
  [X2] -> Gain5/1
  [X2] -> X2/1
  Gain12/1 -> Switch1/1
  [X1] -> Add1/1
  Gain5/1 -> Add1/3
  [X3] -> X3/1

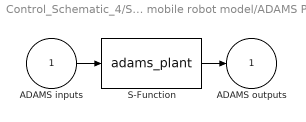
== system Control_Schematic_4/Single mobile robot model/ADAMS Plant ==
  ADAMS inputs : Inport
  S-Function : S-Function  StopFcn=clear mex  FunctionName=adams_plant  Parameters=exevie,exesol,stat,outfil,nampre,o_rate,nam_in,namout,dft,modsim,modani,dt_out,inicmd,exetyp,comtyp,ada_host, workdir,pin_interp_order,pout_extrap_order,pin_extrap_order,pout_interp_order,simulink_lead_cosim  EnableBusSupport=off
  ADAMS outputs : Outport  InitialOutput=0
  wires:
  S-Function/1 -> ADAMS outputs/1
  ADAMS inputs/1 -> S-Function/1
